simulink subsystem "PvtSubSys_LATC"  (R2020b)
settings: Solver=VariableStepAuto  StartTime=0.0  StopTime=10.0  RelTol=1e-3
values from neighbouring files (symbols this model uses):
  P_Global_CharSpd_ms : value not decoded    [PubParsGlobal.sldd]
  P_Global_SteeringAngleRatio : value not decoded    [PubParsGlobal.sldd]
  P_Global_WheelBase_m : value not decoded    [PubParsGlobal.sldd]
  P_LCS_A0_Dis_BP : value not decoded    [SubMdlDD_LATC.sldd]
  P_LCS_A2_Curve_BP : value not decoded    [SubMdlDD_LATC.sldd]
  P_LCS_A2_LatAcc_BP : value not decoded    [SubMdlDD_LATC.sldd]
  P_LCS_A2_Pretime = 0.075    [SubMdlDD_LATC.sldd]
  P_LCS_A2S_FliterTime = 0.5    [SubMdlDD_LATC.sldd]
  P_LCS_AngErrReversSign_SourceSW = 1.0    [SubMdlDD_LATC.sldd]
  P_LCS_AngleErrorReversTorq : value not decoded    [SubMdlDD_LATC.sldd]
  P_LCS_AngleErrorReversTorq_LC_TarAngleBp : value not decoded    [SubMdlDD_LATC.sldd]
  P_LCS_AngleErrorReversTorq_LC_TarAngleFac : value not decoded    [SubMdlDD_LATC.sldd]
  P_LCS_AngleErrorReversTorq_LC_VehSpdBp : value not decoded    [SubMdlDD_LATC.sldd]
  P_LCS_AngleErrorReversTorq_LC_VehSpdVal : value not decoded    [SubMdlDD_LATC.sldd]
  P_LCS_AngleErrorReversTorq_VehSpdBp : value not decoded    [SubMdlDD_LATC.sldd]
  P_LCS_AngleErrorReversTorq_VehSpdFac : value not decoded    [SubMdlDD_LATC.sldd]
  P_LCS_AngleFilterTime = 0.1    [SubMdlDD_LATC.sldd]
  P_LCS_AngleSlope_AES_Active = 0.4 0.4 0.4 0.35 0.35 0.35 0.35 0.35 0.35 0.3 0.3 0.3 0.3 0.3 0.3 0.3 0.3 0.3 0.3 0.4 0.4 0.4 0.35 0.35 0.35 0.35 0.35 0.35 0.3 0.3 0.3 0.3 0.3 0.3 0.3 0.3 0.3 0.3 0.4 0.4 0.4 0.35 0.35 0.35 0.35 0.35 0.35 0.3 0.3 0.3 0.3 0.3 0.3 0.3 0.3 0.3 0.3 0.4 0.4 0.4 0.35 0.35 0.35 0.35 0.35 0.35 0.3 0.3 0.3 0.3 0.3 0.3 0.3 0.3 0.3 0.3 0.4 0.4 0.4 0.35 0.35 0.35 0.35 0.35 0.35 0.3 0.3 0.3 0.3 0.3 0.3 0.3 0.    [SubMdlDD_LATC.sldd]
  P_LCS_AngleSlope_ESS_Add = 1.0 1.0 1.0 1.0 2.0 2.0 2.0 7.0 7.0 7.0 7.0 7.0 7.0 7.0 7.0 7.0 7.0 7.0 7.0 1.0 1.0 1.0 1.0 2.0 2.0 2.0 7.0 7.0 7.0 7.0 7.0 7.0 7.0 7.0 7.0 7.0 7.0 7.0 1.0 1.0 1.0 1.0 2.0 2.0 2.0 7.0 7.0 7.0 7.0 7.0 7.0 7.0 7.0 7.0 7.0 7.0 7.0 1.0 1.0 1.0 1.0 2.0 2.0 2.0 7.0 7.0 7.0 7.0 7.0 7.0 7.0 7.0 7.0 7.0 7.0 7.0 1.0 1.0 1.0 1.0 7.5 7.5 7.5 7.5 7.5 7.5 7.5 7.5 7.5 7.5 7.5 8.0 8.0 8.0 8.0 1.0 1.0 1.0 1.0 7.5    [SubMdlDD_LATC.sldd]
  P_LCS_AngleSlope_LC_Eco = 0.4 0.4 0.4 0.35 0.35 0.35 0.35 0.35 0.35 0.3 0.3 0.3 0.3 0.3 0.3 0.3 0.3 0.3 0.3 0.4 0.4 0.4 0.35 0.35 0.35 0.35 0.35 0.35 0.3 0.3 0.3 0.3 0.3 0.3 0.3 0.3 0.3 0.3 0.4 0.4 0.4 0.35 0.35 0.35 0.35 0.35 0.35 0.3 0.3 0.3 0.3 0.3 0.3 0.3 0.3 0.3 0.3 0.4 0.4 0.4 0.35 0.35 0.35 0.35 0.35 0.35 0.3 0.3 0.3 0.3 0.3 0.3 0.3 0.3 0.3 0.3 0.4 0.4 0.4 0.35 0.35 0.35 0.35 0.35 0.35 0.3 0.3 0.3 0.3 0.3 0.3 0.3 0.    [SubMdlDD_LATC.sldd]
  P_LCS_AngleSlope_LC_Nomal = 0.4 0.4 0.4 0.35 0.35 0.35 0.35 0.35 0.35 0.3 0.3 0.3 0.3 0.3 0.3 0.3 0.3 0.3 0.3 0.4 0.4 0.4 0.35 0.35 0.35 0.35 0.35 0.35 0.3 0.3 0.3 0.3 0.3 0.3 0.3 0.3 0.3 0.3 0.4 0.4 0.4 0.35 0.35 0.35 0.35 0.35 0.35 0.3 0.3 0.3 0.3 0.3 0.3 0.3 0.3 0.3 0.3 0.4 0.4 0.4 0.35 0.35 0.35 0.35 0.35 0.35 0.3 0.3 0.3 0.3 0.3 0.3 0.3 0.3 0.3 0.3 0.4 0.4 0.4 0.35 0.35 0.35 0.35 0.35 0.35 0.3 0.3 0.3 0.3 0.3 0.3 0.3 0.    [SubMdlDD_LATC.sldd]
  P_LCS_AngleSlope_LC_Sport = 0.4 0.4 0.4 0.35 0.35 0.35 0.35 0.35 0.35 0.3 0.3 0.3 0.3 0.3 0.3 0.3 0.3 0.3 0.3 0.4 0.4 0.4 0.35 0.35 0.35 0.35 0.35 0.35 0.3 0.3 0.3 0.3 0.3 0.3 0.3 0.3 0.3 0.3 0.4 0.4 0.4 0.35 0.35 0.35 0.35 0.35 0.35 0.3 0.3 0.3 0.3 0.3 0.3 0.3 0.3 0.3 0.3 0.4 0.4 0.4 0.35 0.35 0.35 0.35 0.35 0.35 0.3 0.3 0.3 0.3 0.3 0.3 0.3 0.3 0.3 0.3 0.4 0.4 0.4 0.35 0.35 0.35 0.35 0.35 0.35 0.3 0.3 0.3 0.3 0.3 0.3 0.3 0.    [SubMdlDD_LATC.sldd]
  P_LCS_AngleSlope_LCK = 0.4 0.4 0.4 0.4 0.4 0.4 0.4 0.4 0.4 0.4 0.4 0.4 0.4 0.4 0.4 0.4 0.4 0.4 0.4 0.4 0.4 0.4 0.4 0.4 0.4 0.4 0.4 0.4 0.4 0.4 0.4 0.4 0.4 0.4 0.4 0.4 0.4 0.4 0.4 0.4 0.4 0.4 0.4 0.4 0.4 0.4 0.4 0.4 0.4 0.4 0.4 0.4 0.4 0.4 0.4 0.4 0.4 0.4 0.4 0.4 0.4 0.4 0.4 0.4 0.4 0.4 0.4 0.4 0.4 0.4 0.4 0.4 0.4 0.4 0.4 0.4 0.4 0.4 0.4 0.4 0.4 0.4 0.4 0.4 0.4 0.4 0.4 0.4 0.4 0.4 0.4 0.4 0.4 0.4 0.4 0.4 0.4 0.4 0.4 0.4    [SubMdlDD_LATC.sldd]
  P_LCS_AngleSlope_LCKIE = 0.4 0.4 0.4 0.4 0.4 0.4 0.4 0.4 0.4 0.4 0.4 0.4 0.4 0.4 0.4 0.4 0.4 0.4 0.4 0.4 0.4 0.4 0.4 0.4 0.4 0.4 0.4 0.4 0.4 0.4 0.4 0.4 0.4 0.4 0.4 0.4 0.4 0.4 0.4 0.4 0.4 0.4 0.4 0.4 0.4 0.4 0.4 0.4 0.4 0.4 0.4 0.4 0.4 0.4 0.4 0.4 0.4 0.4 0.4 0.4 0.4 0.4 0.4 0.4 0.4 0.4 0.4 0.4 0.4 0.4 0.4 0.4 0.4 0.4 0.4 0.4 0.4 0.4 0.4 0.4 0.4 0.4 0.4 0.4 0.4 0.4 0.4 0.4 0.4 0.4 0.4 0.4 0.4 0.4 0.4 0.4 0.4 0.4 0.4 0.4    [SubMdlDD_LATC.sldd]
  P_LCS_AngleSlope_LKA = 0.2 0.2 0.3 0.4 0.4 0.4 0.4 0.4 0.4 0.4 0.4 0.4 0.4 0.4 0.4 0.4 0.4 0.4 0.4 0.2 0.2 0.3 0.4 0.4 0.4 0.4 0.4 0.4 0.4 0.4 0.4 0.4 0.4 0.4 0.4 0.4 0.4 0.4 0.2 0.2 0.3 0.4 0.4 0.4 0.4 0.4 0.4 0.4 0.4 0.4 0.4 0.4 0.4 0.4 0.4 0.4 0.4 0.2 0.2 0.3 0.4 0.4 0.4 0.4 0.4 0.4 0.4 0.4 0.4 0.4 0.4 0.4 0.4 0.4 0.4 0.4 0.2 0.2 0.3 0.4 0.4 0.4 0.4 0.4 0.4 0.4 0.4 0.4 0.4 0.4 0.4 0.4 0.4 0.4 0.4 0.2 0.2 0.3 0.4 0.4    [SubMdlDD_LATC.sldd]
  P_LCS_AngleSlope_Spd_BP : value not decoded    [SubMdlDD_LATC.sldd]
  P_LCS_CurAngleFiltEnable = 1    [SubMdlDD_LATC.sldd]
  P_LCS_CurAngleFilterFC = 2.0    [SubMdlDD_LATC.sldd]
  P_LCS_CurentOffset_LimitValue = 0.001    [SubMdlDD_LATC.sldd]
  P_LCS_CurOffset_SterAngleSpd_Enable = 0.0    [SubMdlDD_LATC.sldd]
  P_LCS_CurOffset_SterAngleSpd_LimitValue = 6.0    [SubMdlDD_LATC.sldd]
  P_LCS_CurOffset_VehicleSpd_LimitValue = 7.0    [SubMdlDD_LATC.sldd]
  P_LCS_CurOffsetA2_Enable = 0.0    [SubMdlDD_LATC.sldd]
  P_LCS_CurOffsetA2_FliterTime = 0.2    [SubMdlDD_LATC.sldd]
  P_LCS_DeltaEps_SpdBp : value not decoded    [SubMdlDD_LATC.sldd]
  P_LCS_DeltaEps_TimeVal : value not decoded    [SubMdlDD_LATC.sldd]
  P_LCS_DesAngle_DelaySample : value not decoded    [SubMdlDD_LATC.sldd]
  P_LCS_DetNoOverRide_DrvTrq_TH : value not decoded    [SubMdlDD_LATC.sldd]
  P_LCS_DetOverRide_DrvTrq_TH : value not decoded    [SubMdlDD_LATC.sldd]
  P_LCS_EPSNotActiveSpdValue = 3.0    [SubMdlDD_LATC.sldd]
  P_LCS_ESS_AngleSlope_Limit = 2.9    [SubMdlDD_LATC.sldd]
  P_LCS_ESS_LogicTest_Enable = 1.0    [SubMdlDD_LATC.sldd]
  P_LCS_ESS_MaxTorqSlope : value not decoded    [SubMdlDD_LATC.sldd]
  P_LCS_ESS_NotActiveFlgDelayTime = 0.0    [SubMdlDD_LATC.sldd]
  P_LCS_ESS_NotActiveFlgDelayTimeSW = 0.0    [SubMdlDD_LATC.sldd]
  P_LCS_ESS_SteerAngleErr : value not decoded    [SubMdlDD_LATC.sldd]
  P_LCS_ESS_SteerAngleFilterTime = 0.2    [SubMdlDD_LATC.sldd]
  P_LCS_ESS_TarAngleFilterTime = 0.2    [SubMdlDD_LATC.sldd]
  P_LCS_ESSAngleSW2 = 0.0    [SubMdlDD_LATC.sldd]
  P_LCS_ESSOverrideTime1 = 0.06    [SubMdlDD_LATC.sldd]
  P_LCS_ESSOverrideTime2 = 0.06    [SubMdlDD_LATC.sldd]
  P_LCS_ESSOverrideTime3 = 0.06    [SubMdlDD_LATC.sldd]
  P_LCS_ESSOverrideValue1 = 20.0    [SubMdlDD_LATC.sldd]
  P_LCS_ESSOverrideValue2 = 20.0    [SubMdlDD_LATC.sldd]
  P_LCS_FF_A0_Speed_Factor : value not decoded    [SubMdlDD_LATC.sldd]
  P_LCS_FF_A0_Torq : value not decoded    [SubMdlDD_LATC.sldd]
  P_LCS_FF_EnableSpd = 5.0    [SubMdlDD_LATC.sldd]
  P_LCS_FF_LCRevs_SpdBP : value not decoded    [SubMdlDD_LATC.sldd]
  P_LCS_FF_LCRevs_SpdVal : value not decoded    [SubMdlDD_LATC.sldd]
  P_LCS_FF_LCRevs_TimeBP : value not decoded    [SubMdlDD_LATC.sldd]
  P_LCS_FF_LCRevs_TimeFacVal : value not decoded    [SubMdlDD_LATC.sldd]
  P_LCS_FF_Param_CurveBp : value not decoded    [SubMdlDD_LATC.sldd]
  P_LCS_FF_Param_CurveFac : value not decoded    [SubMdlDD_LATC.sldd]
  P_LCS_FF_Speed_Bp : value not decoded    [SubMdlDD_LATC.sldd]
  P_LCS_FF_Speed_Factor : value not decoded    [SubMdlDD_LATC.sldd]
  P_LCS_FF_TarAngleTorq_Bp : value not decoded    [SubMdlDD_LATC.sldd]
  P_LCS_FF_TarAngleTorq_Factor : value not decoded    [SubMdlDD_LATC.sldd]
  P_LCS_FFW_Torq_AngleBp : value not decoded    [SubMdlDD_LATC.sldd]
  P_LCS_FFW_Torq_SpdBp : value not decoded    [SubMdlDD_LATC.sldd]
  P_LCS_FFW_Torq_V71 : value not decoded    [SubMdlDD_LATC.sldd]
  P_LCS_FFWSwitch : value not decoded    [SubMdlDD_LATC.sldd]
  P_LCS_IN_Offset_Test_SW = 0.0    [SubMdlDD_LATC.sldd]
  P_LCS_IN_Offset_Test_Value = 0.0    [SubMdlDD_LATC.sldd]
  P_LCS_LatAcc2CurveSW = 0.0    [SubMdlDD_LATC.sldd]
  P_LCS_LC_Complete_PreDisFac : value not decoded    [SubMdlDD_LATC.sldd]
  P_LCS_LCK_preDis_Nomal : value not decoded    [SubMdlDD_LATC.sldd]
  P_LCS_MaxTorqSlope : value not decoded    [SubMdlDD_LATC.sldd]
  P_LCS_NoOverRideTime_TH_s : value not decoded    [SubMdlDD_LATC.sldd]
  P_LCS_Offset_FliterTime = 2.0    [SubMdlDD_LATC.sldd]
  P_LCS_OverRideDetect_enable : value not decoded    [SubMdlDD_LATC.sldd]
  P_LCS_OverRideTime_TH_s : value not decoded    [SubMdlDD_LATC.sldd]
  P_LCS_PID_A0_BP : value not decoded    [SubMdlDD_LATC.sldd]
  P_LCS_PID_A0_FF_SW = 0.0    [SubMdlDD_LATC.sldd]
  P_LCS_PID_A0_P : value not decoded    [SubMdlDD_LATC.sldd]
  P_LCS_PID_AngErrFacBp : value not decoded    [SubMdlDD_LATC.sldd]
  P_LCS_PID_AngErrFacBp_P : value not decoded    [SubMdlDD_LATC.sldd]
  P_LCS_PID_AngErrFacVal : value not decoded    [SubMdlDD_LATC.sldd]
  P_LCS_PID_AngErrFacVal_P : value not decoded    [SubMdlDD_LATC.sldd]
  P_LCS_PID_DisableKi_CurveVal = 0.003    [SubMdlDD_LATC.sldd]
  P_LCS_PID_DrvTorqFacBp : value not decoded    [SubMdlDD_LATC.sldd]
  P_LCS_PID_DrvTorqFacVal : value not decoded    [SubMdlDD_LATC.sldd]
  P_LCS_PID_Ki_TarAng_ESS : value not decoded    [SubMdlDD_LATC.sldd]
  P_LCS_PID_Kp_TarAng_ESS : value not decoded    [SubMdlDD_LATC.sldd]
  P_LCS_PID_Kp_TarAng_ESS2 : value not decoded    [SubMdlDD_LATC.sldd]
  P_LCS_PID_Kp_TarTorq_ESS : value not decoded    [SubMdlDD_LATC.sldd]
  P_LCS_PID_Param_CurveBp : value not decoded    [SubMdlDD_LATC.sldd]
  P_LCS_PID_Param_CurveFac : value not decoded    [SubMdlDD_LATC.sldd]
  P_LCS_PID_Param_GainSwitch : value not decoded    [SubMdlDD_LATC.sldd]
  P_LCS_PID_Param_Kd : value not decoded    [SubMdlDD_LATC.sldd]
  P_LCS_PID_Param_KdFilterTime : value not decoded    [SubMdlDD_LATC.sldd]
  P_LCS_PID_Param_Ki : value not decoded    [SubMdlDD_LATC.sldd]
  P_LCS_PID_Param_KiFreaseWhenLC_Enable : value not decoded    [SubMdlDD_LATC.sldd]
  P_LCS_PID_Param_Kp : value not decoded    [SubMdlDD_LATC.sldd]
  P_LCS_PID_Param_Speed_Adapt : value not decoded    [SubMdlDD_LATC.sldd]
  P_LCS_PID_Param_Speed_Factor_D : value not decoded    [SubMdlDD_LATC.sldd]
  P_LCS_PID_Param_Speed_Factor_I : value not decoded    [SubMdlDD_LATC.sldd]
  P_LCS_PID_Param_Speed_Factor_P : value not decoded    [SubMdlDD_LATC.sldd]
  P_LCS_PID_Param_SteerWheelAngle_Adapt : value not decoded    [SubMdlDD_LATC.sldd]
  P_LCS_PID_Param_SteerWheelAngle_Factor_D : value not decoded    [SubMdlDD_LATC.sldd]
  P_LCS_PID_Param_SteerWheelAngle_Factor_P : value not decoded    [SubMdlDD_LATC.sldd]
  P_LCS_PID_Param_SteerWheelSpd_Adapt : value not decoded    [SubMdlDD_LATC.sldd]
  P_LCS_PID_Param_SteerWheelSpd_Factor_D : value not decoded    [SubMdlDD_LATC.sldd]
  P_LCS_PID_Param_SteerWheelSpd_Factor_P : value not decoded    [SubMdlDD_LATC.sldd]
  P_LCS_PID_SteerAngSpdLim : value not decoded    [SubMdlDD_LATC.sldd]
  P_LCS_preDis_AES_Fac = 0.0 0.0 0.0 0.0 -0.1 -0.1 -0.1 -0.1 -0.1 -0.1 0.1 0.1 0.1 0.2 0.2 0.2 0.2 0.2 0.2 0.0 0.0 0.0 0.0 -0.1 -0.1 -0.1 -0.1 -0.1 -0.1 0.1 0.1 0.1 0.2 0.2 0.2 0.2 0.2 0.2 0.0 0.0 0.0 0.0 -0.1 -0.1 -0.1 -0.1 -0.1 -0.1 0.1 0.1 0.1 0.2 0.2 0.2 0.2 0.2 0.2 0.0 0.0 0.0 0.0 -0.1 -0.1 -0.1 -0.1 -0.1 -0.1 0.1 0.1 0.1 0.2 0.2 0.2 0.2 0.2 0.2 0.0 0.0 0.0 0.0 -0.1 -0.1 -0.1 -0.1 -0.1 -0.1 0.2 0.2 0.2 0.35 0.35 0.35    [SubMdlDD_LATC.sldd]
  P_LCS_preDis_LC_Eco_Fac = 0.0 0.0 0.0 0.0 0.25 0.3 0.3 0.3 0.35 0.35 0.45 0.45 0.45 0.55 0.55 0.55 0.55 0.55 0.55 0.0 0.0 0.0 0.0 0.25 0.3 0.3 0.3 0.35 0.35 0.45 0.45 0.45 0.55 0.55 0.55 0.55 0.55 0.55 0.0 0.0 0.0 0.0 0.25 0.3 0.3 0.3 0.35 0.35 0.45 0.45 0.45 0.55 0.55 0.55 0.55 0.55 0.55 0.0 0.0 0.0 0.0 0.25 0.3 0.3 0.3 0.35 0.35 0.45 0.45 0.45 0.55 0.55 0.55 0.55 0.55 0.55 0.0 0.0 0.0 0.0 0.25 0.3 0.3 0.3 0.35 0.35 0.55    [SubMdlDD_LATC.sldd]
  P_LCS_preDis_LC_Fac = 0.0 0.0 0.0 0.0 -0.1 -0.1 -0.1 -0.1 -0.1 -0.1 0.1 0.1 0.1 0.2 0.2 0.2 0.2 0.2 0.2 0.0 0.0 0.0 0.0 -0.1 -0.1 -0.1 -0.1 -0.1 -0.1 0.1 0.1 0.1 0.2 0.2 0.2 0.2 0.2 0.2 0.0 0.0 0.0 0.0 -0.1 -0.1 -0.1 -0.1 -0.1 -0.1 0.1 0.1 0.1 0.2 0.2 0.2 0.2 0.2 0.2 0.0 0.0 0.0 0.0 -0.1 -0.1 -0.1 -0.1 -0.1 -0.1 0.1 0.1 0.1 0.2 0.2 0.2 0.2 0.2 0.2 0.0 0.0 0.0 0.0 -0.1 -0.1 -0.1 -0.1 -0.1 -0.1 0.2 0.2 0.2 0.35 0.35 0.35    [SubMdlDD_LATC.sldd]
  P_LCS_preDis_LC_Nomal_Fac = 0.0 0.0 0.0 0.0 -0.1 -0.1 -0.1 -0.1 -0.1 -0.1 0.1 0.1 0.1 0.2 0.2 0.2 0.2 0.2 0.2 0.0 0.0 0.0 0.0 -0.1 -0.1 -0.1 -0.1 -0.1 -0.1 0.1 0.1 0.1 0.2 0.2 0.2 0.2 0.2 0.2 0.0 0.0 0.0 0.0 -0.1 -0.1 -0.1 -0.1 -0.1 -0.1 0.1 0.1 0.1 0.2 0.2 0.2 0.2 0.2 0.2 0.0 0.0 0.0 0.0 -0.1 -0.1 -0.1 -0.1 -0.1 -0.1 0.1 0.1 0.1 0.2 0.2 0.2 0.2 0.2 0.2 0.0 0.0 0.0 0.0 -0.1 -0.1 -0.1 -0.1 -0.1 -0.1 0.2 0.2 0.2 0.35 0.35 0.35    [SubMdlDD_LATC.sldd]
  P_LCS_preDis_LC_Sport_Fac = 0.0 0.0 0.0 0.0 -0.1 -0.1 -0.1 -0.1 -0.1 -0.1 0.1 0.1 0.1 0.2 0.2 0.2 0.2 0.2 0.2 0.0 0.0 0.0 0.0 -0.1 -0.1 -0.1 -0.1 -0.1 -0.1 0.1 0.1 0.1 0.2 0.2 0.2 0.2 0.2 0.2 0.0 0.0 0.0 0.0 -0.1 -0.1 -0.1 -0.1 -0.1 -0.1 0.1 0.1 0.1 0.2 0.2 0.2 0.2 0.2 0.2 0.0 0.0 0.0 0.0 -0.1 -0.1 -0.1 -0.1 -0.1 -0.1 0.1 0.1 0.1 0.2 0.2 0.2 0.2 0.2 0.2 0.0 0.0 0.0 0.0 -0.1 -0.1 -0.1 -0.1 -0.1 -0.1 0.2 0.2 0.2 0.35 0.35 0.35    [SubMdlDD_LATC.sldd]
  P_LCS_preDis_LCK_A2Curve_Fac2 : value not decoded    [SubMdlDD_LATC.sldd]
  ... (+20 more)
undefined symbols (not defined in the file or in its folder): P_LCS_A2_CurrentOffsetFliterTime, P_LCS_AngleSlope_ELK, P_LCS_AngleSlope_ESS, P_LCS_AngleSlope_LC_Cancel, P_LCS_AngleSlope_LCK_Curve_Fac, P_LCS_CurSteerAngleOffsetLimit_Low, P_LCS_CurSteerAngleOffsetLimit_Up, P_LCS_DesLaneA0, P_LCS_DesLaneA1, P_LCS_ESS_preDis_Nomal, P_LCS_ESSAngleSW, P_LCS_ESSAngSlope_SW, P_LCS_LATC_Effect, P_LCS_MinTorqSlope, P_LCS_PID_Param_Kifactor, P_LCS_preDis_ELK_Fac, P_LCS_preDis_ESS_Fac, P_LCS_preDis_LCK_A2Curve_Fac, P_LCS_preDis_LCK_Fac, P_LCS_StateActiv_AngleSlope, P_LCS_StateActiveFlg_BP, P_LCS_TorqSlope_AngleErrorBp, P_LCS_TorqSlope_AngleErrorVal, P_LCS_TorqSlope_AngleSpdBp, P_LCS_TorqSlope_AngleSpdVal, P_LCS_TorqSlope_TorqErrorBp, P_LCS_TorqSlope_TorqErrorVal
libraries: simulink x59
(part 3 of 75)

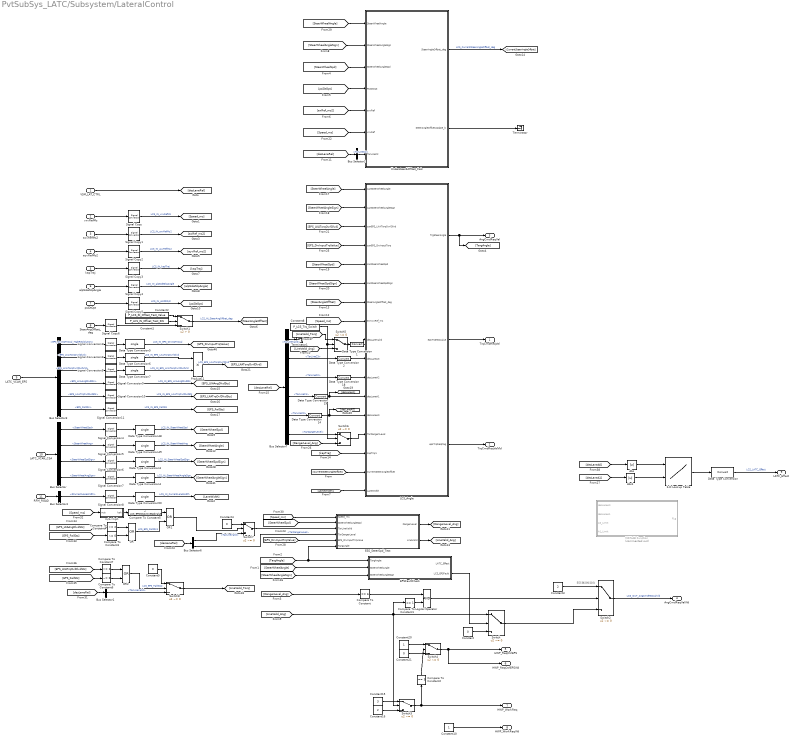
== system PvtSubSys_LATC/Subsystem/LateralControl ==
  note: ESS激活标志位
  VSM_LAT_CTRL : Inport  PortDimensions=1  BusOutputAsStruct=on
  vxvRefMs : Inport  Port=2  OutDataTypeStr=single  PortDimensions=1  BusOutputAsStruct=on
  axvRefMs2 : Inport  Port=3  OutDataTypeStr=single  PortDimensions=1  BusOutputAsStruct=on
  ayvRefMs2 : Inport  Port=4  OutDataTypeStr=single  PortDimensions=1  BusOutputAsStruct=on
  kapTraj : Inport  Port=5  OutDataTypeStr=single  PortDimensions=1  BusOutputAsStruct=on
  alpSideSlipAngle : Inport  Port=6  OutDataTypeStr=single  PortDimensions=1  BusOutputAsStruct=on
  psiDtOpt : Inport  Port=7  OutDataTypeStr=single  PortDimensions=1  BusOutputAsStruct=on
  SteerAngOffset_deg : Inport  Port=8  OutDataTypeStr=single  PortDimensions=1  BusOutputAsStruct=on
  LATC_VCAN_EPS : Inport  Port=9  OutDataTypeStr=Bus: VCAN_EPS_MSG_BUS  PortDimensions=1  BusOutputAsStruct=on
  LATC_VCAN_CSA : Inport  Port=10  OutDataTypeStr=Bus: VCAN_CSA_MSG_BUS  PortDimensions=1  BusOutputAsStruct=on
  RFM_ROAD : Inport  Port=11  OutDataTypeStr=Bus: RFM_ROAD_BUS  PortDimensions=1  BusOutputAsStruct=on
  2-D Lookup Table : Lookup_n-D  BreakpointsForDimension1=P_LCS_DesLaneA0  BreakpointsForDimension2=P_LCS_DesLaneA1  Table=P_LCS_LATC_Effect  ExtrapMethod=Clip  UseLastTableValue=on  InternalRulePriority=Speed  RndMeth=Simplest  InputSameDT=on
      settings: InputPortMap=u0,u1
  Abs : Abs
  Abs1 : Abs
  Bus Selector : BusSelector  OutputSignals=SteerWheelSpd,SteerWheelAng,SteerWheelSpdSign,SteerWheelAngSign
  Bus Selector1 : BusSelector  OutputSignals=TarLineValid
  Bus Selector2 : BusSelector  OutputSignals=TarLineC2
  Bus Selector3 : BusSelector  OutputSignals=EPS_DrvInpTrqVal_HighReslolution,EPS_LKATorqOvrlDlvd,EPS_LKATorqOvrlDlvdVld,EPS_LKAAngDlvdSts,EPS_LKATrqOvlDlvdSts,EPS_FailSts
  Bus Selector4 : BusSelector  OutputSignals=dCurrentLaneWidth
  Bus Selector6 : BusSelector  OutputSignals=TarLineValid,TarDangerLevel
  Bus Selector7 : BusSelector  OutputSignals=TarLineValid,TarLineC3,TarLineC2,TarLineC1,TarLineC0,TarDangerLevel
  Compare To Constant : simulink/Logic and Bit Operations/Compare To Constant  relop===  const=6  OutDataTypeStr=boolean
  Compare To Constant1 : simulink/Logic and Bit Operations/Compare To Constant  relop===  const=1  OutDataTypeStr=boolean
  Compare To Constant2 : simulink/Logic and Bit Operations/Compare To Constant  relop===  const=3  OutDataTypeStr=boolean
  Compare To Constant3 : simulink/Logic and Bit Operations/Compare To Constant  relop=~=  const=0  OutDataTypeStr=boolean
  Compare To Constant4 : simulink/Logic and Bit Operations/Compare To Constant  relop=>=  const=2  OutDataTypeStr=boolean
  Compare To Constant5 : simulink/Logic and Bit Operations/Compare To Constant  relop=<  const=P_LCS_EPSNotActiveSpdValue  OutDataTypeStr=boolean
  Compare To Constant6 : simulink/Logic and Bit Operations/Compare To Constant  relop=~=  const=0  OutDataTypeStr=boolean
  Compare To Constant7 : simulink/Logic and Bit Operations/Compare To Constant  relop=>=  const=2  OutDataTypeStr=boolean
  Constant : Constant  Value=0  OutDataTypeStr=uint8
  Constant1 : Constant  Value=P_LCS_IN_Offset_Test_SW  OutDataTypeStr=uint8
  Constant10 : Constant  OutDataTypeStr=boolean
  Constant15 : Constant  Value=3  OutDataTypeStr=uint8
  Constant16 : Constant  Value=2  OutDataTypeStr=uint8
  Constant2 : Constant  Value=P_LCS_IN_Offset_Test_Value  OutDataTypeStr=single
  Constant20 : Constant  OutDataTypeStr=boolean
  Constant21 : Constant  Value=0  OutDataTypeStr=boolean
  Constant3 : Constant  Value=2  OutDataTypeStr=uint8
  Constant4 : Constant  Value=0  OutDataTypeStr=boolean
  Constant5 : Constant  Value=0  OutDataTypeStr=boolean
  Constant8 : Constant  Value=P_LCS_Trq_Switch  OutDataTypeStr=uint8
  Data Type Conversion{,1..2,14,18..19} (6 alike) : DataTypeConversion
  Data Type Conversion{3..7,48..50} (8 alike) : DataTypeConversion  OutDataTypeStr=single
  EPSFaultCheck : Subsystem
  ESS_SteerSpd_Test : Subsystem
  LCS_Angle : Subsystem
  Logical Operator : Logic  AllPortsSameDT=off  OutDataTypeStr=boolean
  MATLAB Function : MATLAB Function  Commented=on  TreatAsAtomicUnit=on
  OR : Logic  Operator=OR  AllPortsSameDT=off  OutDataTypeStr=boolean
  OR1 : Logic  Operator=OR  AllPortsSameDT=off  OutDataTypeStr=boolean
  OR2 : Logic  Operator=OR  AllPortsSameDT=off  OutDataTypeStr=boolean
  Product11 : Product
  Signal Conversion{1..11} (11 alike) : SignalConversion  OverrideOpt=off
  Signal Copy{,1..6} (7 alike) : SignalConversion  OverrideOpt=off
  Switch{,2..6} (6 alike) : Switch  Criteria=u2 ~= 0
  Switch1 : Switch  Criteria=u2 > Threshold
  Switch7 : Switch  Criteria=u2 ~= 0  Threshold=5
  Switch8 : Switch  Criteria=u2 ~= 0  Threshold=5
  Terminator : Terminator
  Terminator1 : Terminator
  Understeer&Offset_Calc : Subsystem
  m/s->kph : Subsystem
  TrqCmdReqVal : Outport  OutDataTypeStr=single
  TrqCmdReqValVld : Outport  Port=2  OutDataTypeStr=uint8
  AngCmdReqVal : Outport  Port=3  OutDataTypeStr=single
  AngCmdReqValVld : Outport  Port=4
  HWP_ReqCtrlEPS : Outport  Port=5
  HWP_ReqCtrlEPSVld : Outport  Port=6
  HWP_WorkReq : Outport  Port=7
  HWP_WorkReqVld : Outport  Port=8
  LATC_Effect : Outport  Port=9  OutDataTypeStr=single
  wires:
  2-D Lookup Table/1 -> Data Type Conversion/1
  Abs1/1 -> 2-D Lookup Table/2
  Abs/1 -> 2-D Lookup Table/1
  Data Type Conversion/1 -> LATC_Effect/1  "LCS_LATC_Effect"
  [desLaneA0] -> Abs/1
  [desLaneA1] -> Abs1/1
  [LineValid_Torq] -> Switch5/1
  Switch8/1 -> [LineValid_Torq]
  Constant5/1 -> Switch8/1
  OR2/1 -> Switch8/2  "LCS_EPS_FailSts2"
  [EPS_FailSts] -> Compare To Constant6/1
  [EPS_LKATrqOvlDlvdSts] -> Compare To Constant7/1
  Compare To Constant6/1 -> OR2/2
  Compare To Constant7/1 -> OR2/1
  [desLaneRel] -> Bus Selector1/1
  Bus Selector1/1 -> Switch8/3  "<TarLineValid>"
  Signal Conversion11/1 -> [EPS_FailSts]  "LCS_IN_EPS_FailSts"
  Signal Conversion10/1 -> [EPS_LKATrqOvlDlvdSts]  "LCS_IN_EPS_LKATrqOvlDlvdSts"
  Signal Conversion9/1 -> [EPS_LKAAngDlvdSts]  "LCS_IN_EPS_LKAAngDlvdSts"
  Bus Selector3/6 -> Signal Conversion11/1  "<EPS_FailSts>"
  Bus Selector3/5 -> Signal Conversion10/1  "<EPS_LKATrqOvlDlvdSts>"
  Bus Selector3/4 -> Signal Conversion9/1  "<EPS_LKAAngDlvdSts>"
  Signal Conversion3/1 -> Data Type Conversion7/1
  Signal Conversion2/1 -> Data Type Conversion6/1
  Signal Conversion1/1 -> Data Type Conversion5/1
  LATC_VCAN_EPS/1 -> Bus Selector3/1
  Product11/1 -> [EPS_LKATorqOvrlDlvd]  "LCS_EPS_LKATorqOvrlDlvd"
  Bus Selector3/3 -> Signal Conversion3/1  "<EPS_LKATorqOvrlDlvdVld>"
  Bus Selector3/2 -> Signal Conversion2/1  "<EPS_LKATorqOvrlDlvd>"
  Bus Selector3/1 -> Signal Conversion1/1  "<EPS_DrvInpTrqVal_HighReslolution>"
  Data Type Conversion7/1 -> Product11/2  "LCS_IN_EPS_LKATorqOvrlDlvdVld"
  Data Type Conversion6/1 -> Product11/1  "LCS_IN_EPS_LKATorqOvrlDlvd"
  Data Type Conversion5/1 -> [EPS_DrvInputTrqValue]  "LCS_IN_EPS_DrvInpTrqVal"
  [Speed_ms] -> m/s->kph/1(m/s)
  OR1/1 -> Switch7/2
  Compare To Constant3/1 -> OR/2
  OR/1 -> OR1/2  "LCS_EPS_FailSts1"
  m/s->kph/1(kph) -> Compare To Constant5/1
  Compare To Constant5/1 -> OR1/1
  [EPS_LKAAngDlvdSts] -> Compare To Constant4/1
  [EPS_FailSts] -> Compare To Constant3/1
  Compare To Constant4/1 -> OR/1
  Switch7/1 -> ESS_SteerSpd_Test/3(TarLineValid)
  Constant4/1 -> Switch7/1
  [Speed_ms] -> ESS_SteerSpd_Test/1(Speed_ms)
  [DangerLevel_Ang] -> Switch6/3
  Constant8/1 -> Switch5/2, Switch6/2
  [LineValid_Ang] -> Switch5/3
  Switch5/1 -> Data Type Conversion1/1
  [EPS_DrvInputTrqValue] -> ESS_SteerSpd_Test/5(EPS_DrvInputTrqValue)
  Switch6/1 -> LCS_Angle/14(TarDangerlLevel)
  [TargAngle] -> EPSFaultCheck/1(TargAngle), ESS_SteerSpd_Test/6(TargAngle)
  [SteerWheelSpd] -> ESS_SteerSpd_Test/2(SteerWheelAngleSpd)
  [desLaneRel] -> Bus Selector6/1
  Bus Selector6/1 -> Switch7/3  "<TarLineValid>"
  Bus Selector6/2 -> ESS_SteerSpd_Test/4(TarDangerLevel)  "<TarDangerLevel>"
  ESS_SteerSpd_Test/1(DangerLevel) -> [DangerLevel_Ang]
  ESS_SteerSpd_Test/2(LineValid) -> [LineValid_Ang]
  [desLaneRel] -> Bus Selector2/1
  Bus Selector2/1 -> Understeer&Offset_Calc/7(TarLineC2)  "<TarLineC2>"
  Constant3/1 -> Switch2/1
  Switch/1 -> Switch2/3
  Logical Operator/1 -> Switch2/2
  Compare To Constant1/1 -> Logical Operator/2
  Compare To Constant/1 -> Logical Operator/1
  [DangerLevel_Ang] -> Compare To Constant/1
  Signal Conversion8/1 -> Data Type Conversion50/1
  Signal Conversion7/1 -> Data Type Conversion4/1
  Signal Conversion6/1 -> Data Type Conversion3/1
  Signal Conversion5/1 -> Data Type Conversion49/1
  Signal Conversion4/1 -> Data Type Conversion48/1
  Constant2/1 -> Switch1/1
  Constant1/1 -> Switch1/2
  Signal Copy6/1 -> Switch1/3
  [LaneWidth] -> LCS_Angle/17(LaneWidth)
  Switch1/1 -> [SteerAngleOffSet]  "LCS_IN_SteerAngOffset_deg"
  Signal Copy5/1 -> [psiDtOpt]  "LCS_IN_psiDtOpt"
  Signal Copy4/1 -> [alpSideSlipAngle]  "LCS_IN_alpSideSlipAngle"
  Signal Copy3/1 -> [kapTraj]  "LCS_IN_kapTraj"
  Signal Copy2/1 -> [ayvRef_ms2]  "LCS_IN_ayvRefMs2"
  Signal Copy1/1 -> [axRef_ms2]  "LCS_IN_axvRefMs2"
  Signal Copy/1 -> [Speed_ms]  "LCS_IN_vxvRefMs"
  LATC_VCAN_CSA/1 -> Bus Selector/1
  Data Type Conversion50/1 -> [LaneWidth]  "LCS_IN_CurrentLaneWidth"
  Data Type Conversion49/1 -> [SteerWheelAngle]  "LCS_IN_SteerWheelAng"
  Data Type Conversion48/1 -> [SteerWheelSpd]  "LCS_IN_SteerWheelSpd"
  psiDtOpt/1 -> Signal Copy5/1
  alpSideSlipAngle/1 -> Signal Copy4/1
  kapTraj/1 -> Signal Copy3/1
  ayvRefMs2/1 -> Signal Copy2/1
  Bus Selector4/1 -> Signal Conversion8/1  "<dCurrentLaneWidth>"
  RFM_ROAD/1 -> Bus Selector4/1
  Bus Selector/4 -> Signal Conversion7/1  "<SteerWheelAngSign>"
  Bus Selector/3 -> Signal Conversion6/1  "<SteerWheelSpdSign>"
  Bus Selector/1 -> Signal Conversion4/1  "<SteerWheelSpd>"
  Bus Selector/2 -> Signal Conversion5/1  "<SteerWheelAng>"
  SteerAngOffset_deg/1 -> Signal Copy6/1
  axvRefMs2/1 -> Signal Copy1/1
  vxvRefMs/1 -> Signal Copy/1
  Data Type Conversion4/1 -> [SteerWheelAngleSign]  "LCS_IN_SteerWheelAngleSign"
  Data Type Conversion3/1 -> [SteerWheelSpdSign]  "LCS_IN_SteerWheelSpdSign"
  VSM_LAT_CTRL/1 -> [desLaneRel]
  Bus Selector7/3 -> Data Type Conversion18/1  "<TarLineC2>"
  LCS_Angle/1(TrgSteerAngle) -> [TargAngle], AngCmdReqVal/1
  Data Type Conversion14/1 -> [desLaneA0], LCS_Angle/13(desLaneA0)
  [kapTraj] -> LCS_Angle/15(kapTraj1)
  [EPS_DrvInputTrqValue] -> LCS_Angle/4(canEPS_DrvInputTorq)
  [EPS_LKATorqOvrlDlvd] -> LCS_Angle/3(canEPS_LKATorqOvrlDlvd)
  Bus Selector7/2 -> Data Type Conversion2/1  "<TarLineC3>"
  [desLaneRel] -> Bus Selector7/1
  [LineValid_Ang] -> Switch3/2, Switch/1, Compare To Constant1/1
  [SteerAngleOffSet] -> LCS_Angle/7(SteerAngleOffset_deg)
  Bus Selector7/4 -> Data Type Conversion19/1  "<TarLineC1>"
  Bus Selector7/5 -> Data Type Conversion14/1  "<TarLineC0>"
  [SteerWheelSpdSign] -> LCS_Angle/6(canSteerWheelSpdSign)
  [SteerWheelAngleSign] -> LCS_Angle/2(canSteerWheelAngleSign)
  [Speed_ms] -> LCS_Angle/8(eviVxvRef_ms)
  [SteerWheelSpd] -> LCS_Angle/5(canSteerWheelSpd)
  [SteerWheelAngle] -> LCS_Angle/1(canSteerWheelAngle)
  Bus Selector7/1 -> Terminator1/1  "<TarLineValid>"
  Bus Selector7/6 -> Switch6/1  "<TarDangerLevel>"
  Constant10/1 -> HWP_WorkReqVld/1
  Constant16/1 -> Switch3/3
  Switch4/1 -> HWP_ReqCtrlEPSVld/1, HWP_ReqCtrlEPS/1
  Constant15/1 -> Switch3/1
  Compare To Constant2/1 -> Switch4/2
  Constant20/1 -> Switch4/1
  Constant21/1 -> Switch4/3
  Switch3/1 -> HWP_WorkReq/1, Compare To Constant2/1
  Data Type Conversion18/1 -> LCS_Angle/11(desLaneA2)
  Data Type Conversion19/1 -> [desLaneA1], LCS_Angle/12(desLaneA1)
  Switch2/1 -> AngCmdReqValVld/1  "LCS_OUT_AngCmdReqValVld"
  Constant/1 -> Switch/3
  [SteerWheelAngle] -> EPSFaultCheck/2(SteerWheelAngle)
  [SteerWheelAngleSign] -> EPSFaultCheck/3(SteerWheelAngleSign)
  EPSFaultCheck/2(LCS_EPSFault) -> Switch/2
  Data Type Conversion2/1 -> LCS_Angle/10(desLaneA3)
  [Speed_ms] -> Understeer&Offset_Calc/6(vxvRef)
  [SteerWheelAngle] -> Understeer&Offset_Calc/1(SteerWheelAngle)
  [psiDtOpt] -> Understeer&Offset_Calc/4(PsiDtOpt)
  Understeer&Offset_Calc/1(SteerAngleOffset_deg) -> [CurrentSteerAngleOffset]  "LCS_CurrentSteerAngleOffset_deg"
  [axRef_ms2] -> Understeer&Offset_Calc/5(axvRef)
  [SteerWheelSpd] -> Understeer&Offset_Calc/3(SteerWheelAngleSpd)
  [SteerWheelAngleSign] -> Understeer&Offset_Calc/2(SteerWheelAngleSign)
  Understeer&Offset_Calc/2(SteerAngleOffsetUpdate_b) -> Terminator/1
  [CurrentSteerAngleOffset] -> LCS_Angle/16(CurrentSteerAngleOffset)
  Data Type Conversion1/1 -> LCS_Angle/9(desLaneValid)
  LCS_Angle/3(epsTrqReqFlag) -> TrqCmdReqValVld/1
  LCS_Angle/2(epsTrqReqValue) -> TrqCmdReqVal/1
